simulink model "ModelValidation_ExampleII"  (Simulink 2.20)
settings: Solver=ode4  StartTime=0.0  StopTime=3600  FixedStep=0.0025  RelTol=1e-3  AbsTol=1e-6
libraries: DABLib x3
settings Model: ConsistencyChecking=off  RTWPlaceOutputsASAP=off

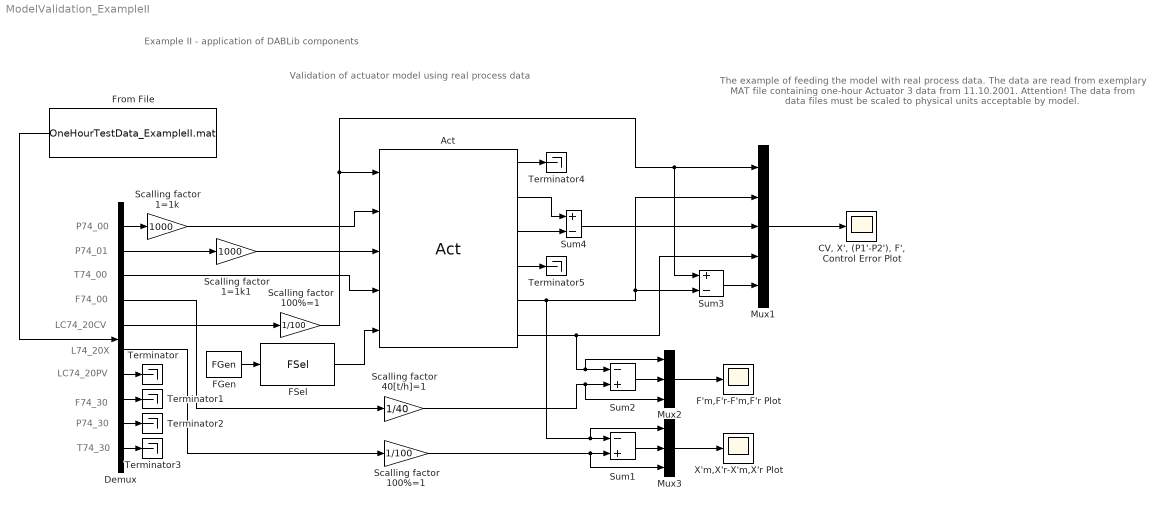
== system ModelValidation_ExampleII ==
  note: Validation of actuator model using real process data
  note: Example II - application of DABLib components
  note: P74_00
  note: P74_01
  note: T74_00
  note: F74_00
  note: LC74_20CV
  note: L74_20X
  note: LC74_20PV
  note: F74_30
  note: P74_30
  note: T74_30
  note: The example of feeding the model with real process data.
      | The data are read from exemplary MAT file containing one-hour Actuator 3 data from 11.10.2001.
      | Attention! The data from data files must be scaled to physical units acceptable by model.
  Act : DABLib/Act  Dist=off
  "CV, X', (P1'-P2'), F', Control Error Plot" : Scope
      settings: TickLabels=on  TimeRange=120  YMin=-0.2  YMax=1  SaveToWorkspace=off  SaveName=ScopeData  LimitMaxRows=off  SampleInput=on  SampleTime=0.1
  Demux : Demux  Outputs=10
  F'm,F'r-F'm,F'r Plot : Scope
      settings: TickLabels=on  TimeRange=120  YMin=-0.2  YMax=1  SaveToWorkspace=off  SaveName=ScopeData  LimitMaxRows=off  SampleInput=on  SampleTime=0.1
  FGen : DABLib/FGen  From=15  To=inf  MFS=0.1  FDT=0  FSD=1
  FSel : DABLib/FSel  FSel=NO FAULT
  From File : FromFile  Orientation=left  FileName=OneHourTestData_ExampleII.mat
  Mux1 : Mux  Inputs=5
  Mux2 : Mux  Inputs=3
  Mux3 : Mux  Inputs=3
  Scalling factor 100%=1 : Gain  Gain=1/100
  "Scalling factor 100%=1 " : Gain  Gain=1/100
  Scalling factor 1=1k : Gain  Gain=1000
  Scalling factor 1=1k1 : Gain  Gain=1000
  Scalling factor 40[t/h]=1 : Gain  Gain=1/40
  Sum1 : Sum  Inputs=-+
  Sum2 : Sum  Inputs=-+
  Sum3 : Sum  Inputs=+-
  Sum4 : Sum  Inputs=+-
  Terminator{,1..5} (6 alike) : Terminator
  X'm,X'r-X'm,X'r Plot : Scope
      settings: TickLabels=on  TimeRange=120  YMin=-0.2  YMax=1  SaveToWorkspace=off  SaveName=ScopeData  LimitMaxRows=off  SampleInput=on  SampleTime=0.1
  wires:
  FGen/1 -> FSel/1
  FSel/1 -> Act/5
  Act/4 -> Terminator5/1
  Act/1 -> Terminator4/1
  From File/1 -> Demux/1
  Demux/10 -> Terminator3/1
  Demux/9 -> Terminator2/1
  Demux/8 -> Terminator1/1
  Demux/7 -> Terminator/1
  Mux1/1 -> "CV, X', (P1'-P2'), F', Control Error Plot"/1
  Sum4/1 -> Mux1/3
  Sum3/1 -> Mux1/5
  Act/2 -> Sum4/1
  Act/3 -> Sum4/2
  Act/6 -> Mux1/4, Sum2/1, Mux2/1
  Act/5 -> Mux1/2, Sum3/2, Sum1/1, Mux3/1
  Mux2/1 -> F'm,F'r-F'm,F'r Plot/1
  Sum2/1 -> Mux2/2
  Sum1/1 -> Mux3/2
  Mux3/1 -> X'm,X'r-X'm,X'r Plot/1
  Scalling factor 100%=1/1 -> Act/1, Mux1/1, Sum3/1
  Demux/5 -> Scalling factor 100%=1/1
  Demux/4 -> Scalling factor 40[t/h]=1/1
  Demux/6 -> "Scalling factor 100%=1 "/1
  Demux/1 -> Scalling factor 1=1k/1
  Demux/2 -> Scalling factor 1=1k1/1
  Scalling factor 1=1k/1 -> Act/2
  Scalling factor 1=1k1/1 -> Act/3
  Scalling factor 40[t/h]=1/1 -> Sum2/2, Mux2/3
  "Scalling factor 100%=1 "/1 -> Sum1/2, Mux3/3
  Demux/3 -> Act/4
